simulink model "TrafficLight"  (R2017b)
settings: Solver=FixedStepDiscrete  StartTime=0.0  StopTime=inf  RelTol=1e-3
settings Model: Creator=Hady Sallam  LastModifiedBy=Hady Sallam
settings OptimizationCC: DefaultParameterBehavior=Inlined  PassReuseOutputArgsAs=Individual arguments
settings DebuggingCC: ParameterTunabilityLossMsg=error
settings SFSimCC: MATLABDynamicMemAlloc=off
settings RTWCC: SystemTargetFile=ert.tlc  GenCodeOnly=on  TemplateMakefile=ert_default_tmf  GenerateReport=on  IncludeHyperlinkInReport=on  LaunchReport=on  GenerateTraceInfo=on  GenerateTraceReport=on  GenerateTraceReportSl=on  GenerateTraceReportSf=on  GenerateTraceReportEml=on
settings CodeAppCC: ForceParamTrailComments=on  IgnoreCustomStorageClasses=off  OperatorAnnotations=on  SimulinkDataObjDesc=on  SFDataObjDesc=on  InsertBlockDesc=on
settings ERTTargetCC: TargetLangStandard=C99 (ISO)  GenerateSampleERTMain=on  InlinedParameterPlacement=NonHierarchical  ERTCustomFileTemplate=example_file_process.tlc  EnableUserReplacementTypes=on

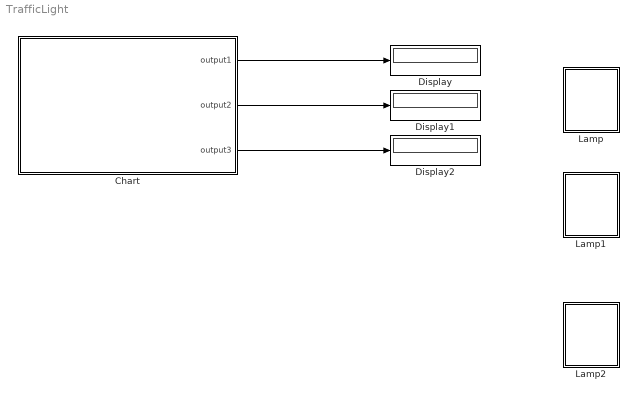
== system TrafficLight ==
  Chart : Stateflow chart  TreatAsAtomicUnit=on
  Display : Display
  Display1 : Display
  Display2 : Display
  Lamp : Subsystem  DialogController=hmiCreateDDGDialog  IsWebBlock=on  mask(MWDashboardBlock){webBlockId=d5f7fba4-ea9d-4eee-ab69-fb771c8b9935, webBlockType=lamp, ShowInLibBrowser=on, ShowInitialText=on, HMISrcModelName=tryStateFlow}
      mask prompts: webBlockType "WebBlock Type"; HMISrcModelName "Source Model"
      mask help: SimulinkHMI:dialogs:LampDialogDesc
      mask Help: helpview([docroot '/mapfiles/simulink.map'], 'hmi_lamp')
      mask Display:
      | if strcmp(get_param(bdroot(gcb),'BlockDiagramType'), 'library')
      |     image([(matlabroot) '/toolbox/simulink/hmi/icons/Lamp.png']);
      | end
  Lamp1 : Subsystem  DialogController=hmiCreateDDGDialog  IsWebBlock=on  mask(MWDashboardBlock){webBlockId=57f74f93-a7a6-4f9f-add1-f2c36f6759ce, webBlockType=lamp, ShowInLibBrowser=on, ShowInitialText=on, HMISrcModelName=tryStateFlow}
      mask prompts: webBlockType "WebBlock Type"; HMISrcModelName "Source Model"
      mask help: SimulinkHMI:dialogs:LampDialogDesc
      mask Help: helpview([docroot '/mapfiles/simulink.map'], 'hmi_lamp')
      mask Display:
      | if strcmp(get_param(bdroot(gcb),'BlockDiagramType'), 'library')
      |     image([(matlabroot) '/toolbox/simulink/hmi/icons/Lamp.png']);
      | end
  Lamp2 : Subsystem  DialogController=hmiCreateDDGDialog  IsWebBlock=on  mask(MWDashboardBlock){webBlockId=a1a09b40-4bf9-4379-93d8-d37bea51bffc, webBlockType=lamp, ShowInLibBrowser=on, ShowInitialText=on, HMISrcModelName=tryStateFlow}
      mask prompts: webBlockType "WebBlock Type"; HMISrcModelName "Source Model"
      mask help: SimulinkHMI:dialogs:LampDialogDesc
      mask Help: helpview([docroot '/mapfiles/simulink.map'], 'hmi_lamp')
      mask Display:
      | if strcmp(get_param(bdroot(gcb),'BlockDiagramType'), 'library')
      |     image([(matlabroot) '/toolbox/simulink/hmi/icons/Lamp.png']);
      | end
  wires:
  Chart/1(output1) -> Display/1
  Chart/2(output2) -> Display1/1
  Chart/3(output3) -> Display2/1

== system TrafficLight/Lamp ==

== system TrafficLight/Lamp1 ==

== system TrafficLight/Lamp2 ==

== stateflow chart TrafficLight/Chart ==
  state du_1
    output1 = 1;
    output2 = 0;
    output3 = 0;
  state du_
    output1 = 0;
    output2 = 1;
    output3 = 0;
  state du_2
    output1 = 0;
    output2 = 0;
    output3 = 1;
  (default) -> state14
  state14 -> state16 : after(3,sec)
  state16 -> state18 : after(3,sec)
  state18 -> state14 : after(3, sec)
  data: output1 output double; output2 output double; output3 output double
